simulink model "solution_imageFeatures_exercise"  (R2021b)
settings: Solver=VariableStepAuto  StartTime=0.0  StopTime=10  RelTol=1e-3
InitFcn:
  | initVars
undefined symbols (not defined in the file or in its folder): gray, Rec, SDTV
libraries: visionconversions x2, dspvision x1, visiongeotforms x1
settings Model: Creator=lipingw  LastModifiedBy=mmordeka
settings DebuggingCC: ParameterPrecisionLossMsg=none

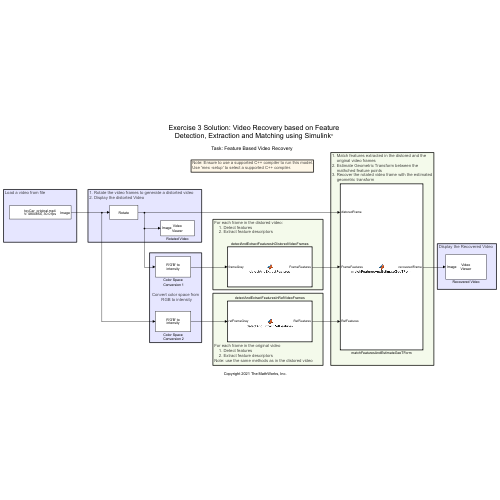
[thumbnail: Simulink's stored preview of the top-level diagram]
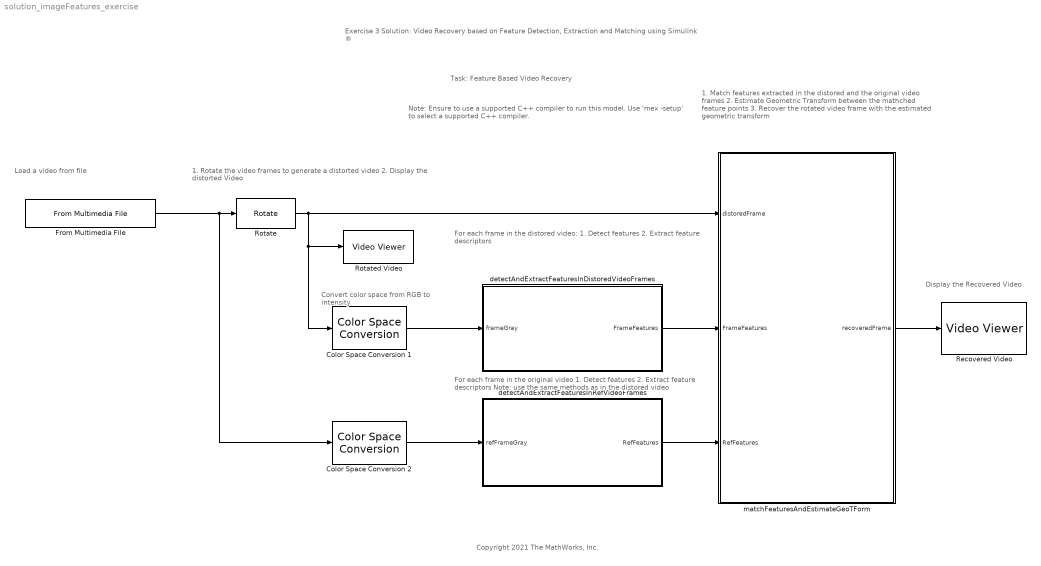
== system solution_imageFeatures_exercise ==
  note: Exercise 3 Solution: Video Recovery based on Feature Detection, Extraction and Matching using Simulink ®
  note: Task: Feature Based Video Recovery
  note: Copyright 2021 The MathWorks, Inc.
  note: Note: Ensure to use a supported C++ compiler to run this model.
      | Use 'mex -setup' to select a supported C++ compiler.
  note: 1. Rotate the video frames to generate a distorted video
      | 2. Display the distorted Video
  note: For each frame in the distored video:
      |     1. Detect features
      |     2. Extract feature descriptors
  note: For each frame in the original video
      |     1. Detect features
      |     2. Extract feature descriptors
      | Note: use the same methods as in the distored video
  note: 1. Match features extracted in the distored and the
      |     original video frames
      | 2. Estimate Geometric Transform between the
      |     mathched feature points
      | 3. Recover the rotated video frame with the estimated
      |     geometric transform
  note: Display the Recovered Video
  note: Convert color space from
      |          RGB to intensity
  note: Load a video from file
  Color Space Conversion 1 : visionconversions/Color Space  Conversion  conversion=Obsolete  conversionActive=R'G'B' to intensity  wp_str=D65  rec=Rec. 601 (SDTV)  sys=1125/60/2:1  imagePorts=One multidimensional signal
  Color Space Conversion 2 : visionconversions/Color Space  Conversion  conversion=Obsolete  conversionActive=R'G'B' to intensity  wp_str=D65  rec=Rec. 601 (SDTV)  sys=1125/60/2:1  imagePorts=One multidimensional signal
  From Multimedia File : dspvision/From Multimedia File  inputFilename=toyCar_original.mp4  readRange=[1 Inf]  loop=on  numPlays=inf  outputStreams=Video only  videoDataType=single  audioDataType=int16  inheritSampleTime=on  userDefinedSampleTime=1/30  noAudioOutput=off  isIntensityVideo=off  fourcc=RGB  colorVideoFormat=One multidimensional signal  outputEOF=off  dataOrg=Column-major  audioFrameSize=1024  computeAudioFrameSize=off  outSamplingMode=Sample based
  Recovered Video : VideoViewer  colormapValue=gray(256)  FigPos=[587 619 691 435]
  Rotate : visiongeotforms/Rotate  outSizeR=Expanded to fit rotated input image  src_angle=Specify via dialog  unit_angle=Degrees  angle=rotateAngle  maxAngle=pi  dispImage=Top-left corner  method=Table lookup  fillVal=0  interpMethod=Bilinear  roundingMode=Nearest  overflowMode=on  prodOutputMode=Binary point scaling  prodOutputWordLength=32  prodOutputFracLength=10
  Rotated Video : VideoViewer  colormapValue=gray(256)  FigPos=[2 677 711 568]
  detectAndExtractFeaturesInDistoredVideoFrames : MATLAB Function  TreatAsAtomicUnit=on
  detectAndExtractFeaturesInRefVideoFrames : MATLAB Function  TreatAsAtomicUnit=on
  matchFeaturesAndEstimateGeoTForm : MATLAB Function  TreatAsAtomicUnit=on
  wires:
  Rotate/1 -> matchFeaturesAndEstimateGeoTForm/1(distoredFrame), Rotated Video/1, Color Space Conversion 1/1
  Color Space Conversion 1/1 -> detectAndExtractFeaturesInDistoredVideoFrames/1(frameGray)
  detectAndExtractFeaturesInDistoredVideoFrames/1(FrameFeatures) -> matchFeaturesAndEstimateGeoTForm/2(FrameFeatures)
  From Multimedia File/1 -> Color Space Conversion 2/1, Rotate/1
  Color Space Conversion 2/1 -> detectAndExtractFeaturesInRefVideoFrames/1(refFrameGray)
  detectAndExtractFeaturesInRefVideoFrames/1(RefFeatures) -> matchFeaturesAndEstimateGeoTForm/3(RefFeatures)
  matchFeaturesAndEstimateGeoTForm/1(recoveredFrame) -> Recovered Video/1

== matlab function solution_imageFeatures_exercise/detectAndExtractFeaturesInDistoredVideoFrames ==
  data: frameGray input; FrameFeatures output Bus: FeatureBus; FrameFeaturesTemp parameter
function FrameFeatures = detectAndExtractFeatures(frameGray, FrameFeaturesTemp) %#codegen
    %% Please implement this section    
     % -- Detect feature points in frameGray using the SURF method  
     detectedPoints = detectSURFFeatures(frameGray);
    
     % -- Extract feature descriptors (featureDescriptors) of the detected feature points (points)
     %    with auto selected method
     [featureDescriptors, points] = extractFeatures(frameGray, detectedPoints);
    
    %% Update output FrameFeatures
     maxNumOfOutputFeatures = size(FrameFeaturesTemp.locations,1);
     numDetected = min(points.Count,maxNumOfOutputFeatures); 
     FrameFeaturesTemp.count = numDetected;   
     FrameFeaturesTemp.locations(1:numDetected,:) = points.Location(1:numDetected,:);
     FrameFeaturesTemp.descriptors(1:numDetected,:) = featureDescriptors(1:numDetected,:);
     FrameFeatures = FrameFeaturesTemp;

== matlab function solution_imageFeatures_exercise/matchFeaturesAndEstimateGeoTForm ==
  data: distoredFrame input; FrameFeatures input; RefFeatures input; recoveredFrame output
function recoveredFrame  = matchFeaturesAndEstimateGeoTForm(distoredFrame,FrameFeatures,RefFeatures)  %#codegen
    %% Get descriptors of the matched features 
    refFeatureDescriptors = RefFeatures.descriptors(1:RefFeatures.count,:);
    frameFeatureDescriptors = FrameFeatures.descriptors(1:FrameFeatures.count,:);
    
    %% Please implement this section
     % -- Match Features based on refFeatureDescriptors and frameFeatureDescriptors
     matchFeaturePairs = matchFeatures(refFeatureDescriptors, frameFeatureDescriptors);
       
     % -- Get putatively matched feature points
     matchedRefPoints = RefFeatures.locations(matchFeaturePairs(:, 1), :);
     matchedFramePoints = FrameFeatures.locations(matchFeaturePairs(:, 2), :);
    
     % -- Estimate geometric transformation (tform) between matched feature points
     [tform,~,~] = ...
        estimateGeometricTransform2D(matchedFramePoints,matchedRefPoints,'similarity');
    
    %% Recover the distorted video frame based on the estimated geometric transformation
     outputView = imref2d([480 845]);
     recoveredFrame  = imwarp(distoredFrame,tform,'OutputView',outputView);

== matlab function solution_imageFeatures_exercise/detectAndExtractFeaturesInRefVideoFrames ==
  data: refFrameGray input; RefFeatures output Bus: FeatureBus; RefFeaturesTemp parameter
function RefFeatures = detectAndExtractRefFeatures(refFrameGray, RefFeaturesTemp) %#codegen
   %% Please implement this section 
    % -- Detect feature points in frameGray using the SURF method  
    detectedPoints = detectSURFFeatures(refFrameGray);
    
    % -- Extract feature descriptors (featureDescriptors) of the detected feature points (points)
    %    with auto selected method
    [featureDescriptors, points] = extractFeatures(refFrameGray, detectedPoints);
    
    %% Update output RefFeatures
     maxNumOfOutputFeatures = size(RefFeaturesTemp.locations,1);
     numDetected = min(points.Count,maxNumOfOutputFeatures); 
     RefFeaturesTemp.count = numDetected;   
     RefFeaturesTemp.locations(1:numDetected,:) = points.Location(1:numDetected,:);
     RefFeaturesTemp.descriptors(1:numDetected,:) = featureDescriptors(1:numDetected,:);
     RefFeatures = RefFeaturesTemp;
